simulink model "MFA_sim"  (R2019a)
settings: Solver=ode5  StartTime=0.0  StopTime=100  FixedStep=0.01  RelTol=1e-3
model workspace: external: MAT-File E:\BKel\202\NMDKTM\btl\matlab\matlab.mat (data not in the file)
undefined symbols (not defined in the file or in its folder): sigbuilder_block
settings Model: OrderedModelArguments=off  Creator=khiem  LastModifiedBy=khiem

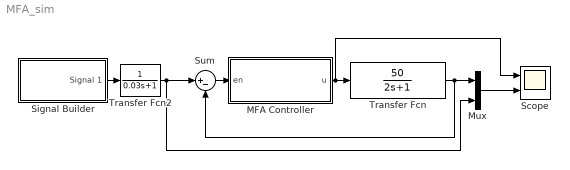
== system MFA_sim ==
  MFA Controller : Subsystem
  Mux : Mux  Inputs=2
  Scope : Scope  NumInputPorts=2
  Signal Builder : Subsystem  Tag=STV Subsys  LoadFcn=sigbuilder_block('load');  StartFcn=sigbuilder_block('start');  StopFcn=sigbuilder_block('stop');  ClipboardFcn=sigbuilder_block('clipboard');  mask(Sigbuilder block){tuvar=[0:10]}
      mask help: Simulink:masks:SigbuilderBlock_MD
      mask init:
      | if ~strcmp(get_param(bdroot(gcbh),'SimulationStatus'),'stopped') tuvar = sigbuilder_block('maskInit'); end
      settings: CopyFcn=sigbuilder_block('copy');  DeleteFcn=sigbuilder_block('delete');  ModelCloseFcn=sigbuilder_block('modelClose');  PreSaveFcn=sigbuilder_block('preSave');  PauseFcn=sigbuilder_block('pause');  ContinueFcn=sigbuilder_block('continue');  NameChangeFcn=sigbuilder_block('namechange');  OpenFcn=sigbuilder_block('open',[437.6 199.2 550.4 400 ]);  CloseFcn=sigbuilder_block('close');
      mask Display: plot(0, 0, 100, 100,[2, 2, 32, 32, 2], [68, 8, 8, 68, 68],[32, 2], [38, 38], [32, 19, 2],[53, 60, 44], [32, 17, 17, 2],[16, 16, 31, 31]);txt = getActiveGroup(gcbh);text(2, 100, txt,'verticalAlignment', 'top');
  Sum : Sum  Inputs=|+-
  Transfer Fcn : TransferFcn  Numerator=[50]  Denominator=[2 1]
  Transfer Fcn2 : TransferFcn  Denominator=[0.03 1]
  wires:
  Sum/1 -> MFA Controller/1(en)
  MFA Controller/1(u) -> Scope/1, Transfer Fcn/1
  Transfer Fcn/1 -> Mux/1, Sum/2
  Mux/1 -> Scope/2
  Signal Builder/1(Signal 1) -> Transfer Fcn2/1
  Transfer Fcn2/1 -> Mux/2, Sum/1

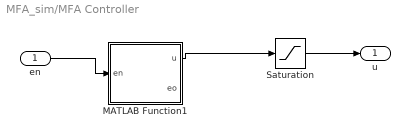
== system MFA_sim/MFA Controller ==
  en : Inport
  MATLAB Function1 : MATLAB Function  TreatAsAtomicUnit=on
  Saturation : Saturate  UpperLimit=1  LowerLimit=-1
  u : Outport
  wires:
  en/1 -> MATLAB Function1/1(en)
  MATLAB Function1/1(u) -> Saturation/1
  Saturation/1 -> u/1

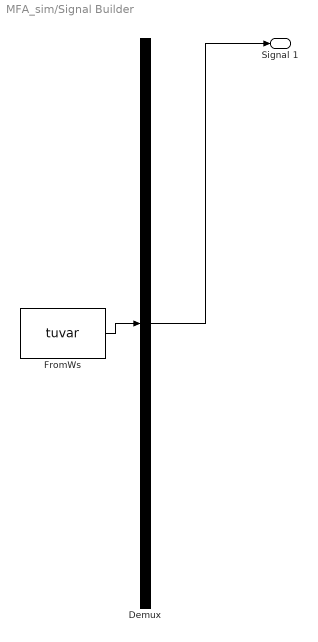
== system MFA_sim/Signal Builder ==
  Demux : Demux  Tag=STV Demux  Outputs=1
  FromWs : FromWorkspace  Tag=STV FromWs  VariableName=tuvar  SampleTime=0
      SigBuilderData=|
      | common.afterFinalStr = 'Extrapolate'
      | common.sampleTime = 0
      | dataSet.timeRange = [0 100]
      | dataSet.name = 'Group 1'
      | sbobj.Groups.Name = 'Group 1'
      | sbobj.Groups.Signals.Name = 'Signal 1'
      | sbobj.Groups.Signals.XData = [0 20 20 40 40 60 60 80 80 100]
      | sbobj.Groups.Signals.YData = [21 21 33.5 33.5 43.5 43.5 22.4 22.4 31.6 31.6]
      | sbobj.Groups.TimeRange = [0 100]
  Signal 1 : Outport  Tag=STV Outport
  wires:
  Demux/1 -> Signal 1/1
  FromWs/1 -> Demux/1

== matlab function MFA_sim/MFA Controller/MATLAB Function1 ==
  settings: updateMethod=DISCRETE
  data: en input; u output; E data_store_memory; e data_store_memory; q data_store_memory; p data_store_memory; w data_store_memory; h data_store_memory; vt data_store_memory; eo output
function [u,eo]= fcn(en)
    global E; global e; global w; global h; global p; global q; global vt;
    N = 8; %N cannot be larger than 20
    Kc = 0.012; eta = 0.2;
    Es = en^2/2;
    if Es > 0
        %% Update error
%         if (en < 0) 
%             en = -en;
%         end
        e = en;
        E(1:N) = [tanh(e/10);E(1:N-1)];

        %% Cal pj and qj
        for j=1:N
            p(j) = w(:,j)' * E + 1;
            q(j) = 1/(1+exp(-p(j)));
%             q(j) = tanh(p(j));
        end

        %% Cal ot and vt
        ot = h'*q + 1;
        vt = Kc * (ot + e);

        %% Cal sum h
        sum_h = 0;
        for k = 1:N
            sum_h = sum_h + h(k);
        end

        %% Update w and h
        for j = 1:N
            for i = 1:N
                w(i,j) = w(i,j) + eta * Kc * e * q(j) * (1 - q(j)) * E(i) * sum_h;
            end
            h(j) = h(j) + eta * Kc * e * q(j);
        end
    end
    %% Output
    eo = e;
    u = vt;
